simulink model "BLDCmotor_FOC_R2017b_fixdt"  (R2025a)
settings: Solver=FixedStepDiscrete  StartTime=0  StopTime=0.5  FixedStep=Ts  MaxStep=1e-6  RelTol=1e-6  AbsTol=1e-6  EnableMultiTasking=on
PreLoadFcn:
  | addpath(pwd);
  | addpath(genpath('01_Libraries'));
  | addpath(genpath('02_Figures'));
  | addpath(genpath('03_CreateParamTable'));
InitFcn:
  | init_model;
values from neighbouring files (symbols this model uses):
  a_cpr = 65535    [init_model.m]
  a_elecAngle = 60    [init_model.m]
  a_elecoffset = a_elecPeriod/12    (= 30)    [init_model.m]
  a_elecPeriod = 360    [init_model.m]
  a_fcpr = 1/65535    (= 1.52590218967e-05)    [init_model.m]
  a_mechoffset = a_elecoffset/n_polePairs    (= 5)    [init_model.m]
  a_phaAdvMax = 25    [init_model.m]
  b_angleMeasEna = 1    [init_model.m]
  b_cruiseCtrlEna = 0    [init_model.m]
  b_diagEna = 0    [init_model.m]
  b_fieldWeakEna = 0    [init_model.m]
  cf_currFilt = 0.692    [init_model.m]
  cf_idKi = Ki / (f_ctrl)    (= 0.00409061543436)    [init_model.m]
  cf_idKp = Kp    (= 0.0523598775598)    [init_model.m]
  cf_iqKi = Ki / (f_ctrl)    (= 0.00409061543436)    [init_model.m]
  cf_iqKiLimProt = 60 / (f_ctrl)    (= 0.00375)    [init_model.m]
  cf_iqKp = Kp    (= 0.0523598775598)    [init_model.m]
  cf_KbLimProt = Simulink.Parameter    [init_model.m]
  cf_nKi = 20.4 / (f_ctrl)    (= 0.001275)    [init_model.m]
  cf_nKiLimProt = 20 / (f_ctrl)    (= 0.00125)    [init_model.m]
  cf_nKp = 1.18    [init_model.m]
  cf_speedCoef = round(f_ctrl * a_mechAngle * (pi/180) * (30/pi))    [init_model.m]
  CTRL_FOC = 2    [init_model.m]
  CTRL_SIN = 1    [init_model.m]
  dV_openRate = 1000 / (f_ctrl)    (= 0.0625)    [init_model.m]
  dz_cntTrnsDetHi = 40    [init_model.m]
  dz_cntTrnsDetLo = 20    [init_model.m]
  ff_gain = ((r_motn / i_sca) * ((GD32_Vd_max_margin) / v_bus))    (= 0.338958333333)    [init_model.m]
  GD32_Vd_max_margin = GD32_Vd_max - V_margin    (= 1627)    [init_model.m]
  GD32_Vq_max_M1 = sqrt(GD32_Vd_max_margin^2 - GD32_Vq_max_XA.^2)    [init_model.m]
  i_max = i_max * i_sca    (= 500)    [init_model.m]
  id_fieldWeakMax = 5 * i_sca    (= 250)    [init_model.m]
  iq_maxSca_M1 = sqrt(1 - iq_maxSca_XA.^2)    [init_model.m]
  mcu_model = GD32F103    (= 1)    [init_model.m]
  n_commAcvLo = 15    [init_model.m]
  n_commDeacvHi = 30    [init_model.m]
  n_cruiseMotTgt = 0    [init_model.m]
  n_fieldWeakAuthHi = 300    [init_model.m]
  n_fieldWeakAuthLo = 100    [init_model.m]
  n_max = 1950    [init_model.m]
  n_polePairs = 6    [init_model.m]
  n_stdStillDet = 3    [init_model.m]
  OPEN_MODE = 0    [init_model.m]
  r_cos_M1 = cos((a_elecAngle_XA + a_elecPeriod/12)*(pi/180))    [init_model.m]
  r_errInpTgtThres = 600    [init_model.m]
  r_fieldWeakHi = 1000    [init_model.m]
  r_fieldWeakLo = 750    [init_model.m]
  r_motn = r_mot/2    (= 0.25)    [init_model.m]
  r_sin3PhaA_M1 = sin3Arm + A*r_sinPhaA_M1    [init_model.m]
  r_sin3PhaB_M1 = sin3Arm + A*r_sinPhaB_M1    [init_model.m]
  r_sin3PhaC_M1 = sin3Arm + A*r_sinPhaC_M1    [init_model.m]
  r_sin_M1 = sin((a_elecAngle_XA + a_elecPeriod/12)*(pi/180))    [init_model.m]
  SPD_MODE = 2    [init_model.m]
  STM32_Vd_max_margin = STM32_Vd_max - V_margin    (= 940)    [init_model.m]
  STM32_Vq_max_M1 = sqrt(STM32_Vd_max_margin^2 - STM32_Vq_max_XA.^2)    [init_model.m]
  t_errDequal = 1.80 * f_ctrl    (= 28800)    [init_model.m]
  t_errQual = 0.24 * f_ctrl    (= 3840)    [init_model.m]
  tgt_scale = 2047    [init_model.m]
  TRQ_MODE = 3    [init_model.m]
  Ts = 5e-6    (= 5e-06)    [init_model.m]
  Ts_ctrl = 6e-5    (= 6e-05)    [init_model.m]
  v_bus = 24    [init_model.m]
  vec_hallToPos = [0 2 0 1 4 3 5 0]    [init_model.m]
  VLT_MODE = 1    [init_model.m]
  z_commutMap_M1 = [-1 -1  0  1  1  0 ... (first row only)    [init_model.m]
  z_ctrlModReq = TRQ_MODE    (= 3)    [init_model.m]
  z_ctrlTypSel = CTRL_FOC    (= 2)    [init_model.m]
  z_maxCntRst = 2000    [init_model.m]
  z_selPhaCurMeasABC = 2    [init_model.m]
undefined symbols (not defined in the file or in its folder): BLDCmotor_FOC_R2017b_fixdt, DiscIntNeverNeededParam, DWORK0, DWORK1, DWORK2, DWORK3, powergui, spspowerguiLib
libraries: BLDC_controller_Lib x18, simulink x13, prociolib x6, eePwmGenerator x6, eePwmGeneratorMultilevel x3, mcbpositiondecoderlib x2, slpidlib x2, spsControlledVoltageSourceLib x1, spsMultimeterLib x1, spsPermanentMagnetSynchronousMachineLib x1, spsUniversalBridgeLib x1, spsVoltageMeasurementLib x1
(part 6 of 6)

== system BLDCmotor_FOC_R2017b_fixdt/BLDC_controller/F05_Field_Oriented_Control/FOC/FOC_Enabled/Torque_Mode/PI_clamp_fixdtFF ==
  err : Inport
  P : Inport  Port=2
  I : Inport  Port=3
  init : Inport  Port=4
  satMax : Inport  Port=5
  satMin : Inport  Port=6
  ext_limProt : Inport  Port=7
  FeedForward : Inport  Port=8
  AND1 : Logic  DisableCoverage=on  Operator=OR  OutDataTypeStr=boolean
  Clamping_circuit : Subsystem
  Constant : Constant  Value=0  OutDataTypeStr=Inherit: Inherit via back propagation
  Divide2 : Product  Inputs=**  RndMeth=Simplest
  Divide5 : Product  Inputs=**  OutDataTypeStr=fixdt(1,16,5)  RndMeth=Simplest  SaturateOnIntegerOverflow=on
  Input : Constant  Value=ff_gain  OutDataTypeStr=fixdt(1,16,12)
  Integrator : Subsystem
  Product : Product  OutDataTypeStr=fixdt(1,16,4)  SaturateOnIntegerOverflow=on
  Saturation_hit : BLDC_controller_Lib/Saturation_hit  SystemSampleTime=-1  VariantActivationTime=update diagram  EmptyChoice=off  PassThrough=off  PassThroughVariantControl=(default)  EmptyChoiceVariantControl=(default)  AllowFlexibleInterface=on  Latency=0  AutoFrameSizeCalculation=off
  Sum1 : Sum  OutDataTypeStr=fixdt(1,16,4)  RndMeth=Simplest  SaturateOnIntegerOverflow=on
  Sum2 : Sum  RndMeth=Simplest  SaturateOnIntegerOverflow=on
  Sum3 : Sum  Inputs=|++  OutDataTypeStr=fixdt(1,16,4)  SaturateOnIntegerOverflow=on
  Switch1 : Switch  Criteria=u2 ~= 0  OutDataTypeStr=Inherit: Inherit via back propagation  RndMeth=Zero  SaturateOnIntegerOverflow=off  InputSameDT=off
  UnitDelay1 : UnitDelay  SampleTime=-1  HasFrameUpgradeWarning=on
      settings: AttributesFormatString=Ini=%<X0>
  out : Outport  VectorParamsAs1DForOutWhenUnconnected=off
  wires:
  I/1 -> Divide2/2
  Sum2/1 -> Switch1/3, Clamping_circuit/1(preIntegrator)
  Sum3/1 -> Saturation_hit/2
  [b_hitSat] -> Clamping_circuit/3(hitSat)
  Saturation_hit/3 -> [b_hitMin]
  P/1 -> Divide5/2
  Saturation_hit/2 -> out/1
  [b_hitMin] -> AND1/2
  init/1 -> Integrator/2(init)
  UnitDelay1/1 -> Switch1/2
  Product/1 -> Sum3/1
  Divide5/1 -> Sum1/1
  satMax/1 -> Saturation_hit/1
  Clamping_circuit/1(Clamp) -> UnitDelay1/1
  FeedForward/1 -> Product/2
  err/1 -> Divide2/1, Divide5/1
  Constant/1 -> Switch1/1
  Saturation_hit/1 -> [b_hitMax]
  Sum1/1 -> Clamping_circuit/2(preSat), Sum3/2
  [b_hitMax] -> AND1/1
  satMin/1 -> Saturation_hit/3
  AND1/1 -> [b_hitSat]
  Switch1/1 -> Integrator/1(u)
  ext_limProt/1 -> Sum2/2
  Divide2/1 -> Sum2/1
  Integrator/1(y) -> Sum1/2
  Input/1 -> Product/1

== system BLDCmotor_FOC_R2017b_fixdt/BLDC_controller/F05_Field_Oriented_Control/FOC/FOC_Enabled/Torque_Mode/Variant Subsystem ==
  note: 1) Add Subsystem or Model blocks as valid variant choices.
      | 2) You cannot connect blocks at this level. At simulation, connectivity is automatically
      | determined, based on the active variant and port name matching.
  GD32F103 : Subsystem  TreatAsAtomicUnit=on  VariantControl=mcu_model == 1
  STM32F103 : Subsystem  TreatAsAtomicUnit=on  VariantControl=mcu_model == 0
  Vd_max_margin : Outport

== system BLDCmotor_FOC_R2017b_fixdt/BLDC_controller/F05_Field_Oriented_Control/FOC/FOC_Enabled/Vd_Calculation/PI_clamp_fixdtFF ==
  err : Inport
  P : Inport  Port=2
  I : Inport  Port=3
  init : Inport  Port=4
  satMax : Inport  Port=5
  satMin : Inport  Port=6
  ext_limProt : Inport  Port=7
  FeedForward : Inport  Port=8
  AND1 : Logic  DisableCoverage=on  Operator=OR  OutDataTypeStr=boolean
  Clamping_circuit : Subsystem
  Constant : Constant  Value=0  OutDataTypeStr=Inherit: Inherit via back propagation
  Divide2 : Product  Inputs=**  RndMeth=Simplest
  Divide5 : Product  Inputs=**  OutDataTypeStr=fixdt(1,16,5)  RndMeth=Simplest  SaturateOnIntegerOverflow=on
  Input : Constant  Value=ff_gain  OutDataTypeStr=fixdt(1,16,12)
  Integrator : Subsystem
  Product : Product  OutDataTypeStr=fixdt(1,16,4)  SaturateOnIntegerOverflow=on
  Saturation_hit : BLDC_controller_Lib/Saturation_hit  SystemSampleTime=-1  VariantActivationTime=update diagram  EmptyChoice=off  PassThrough=off  PassThroughVariantControl=(default)  EmptyChoiceVariantControl=(default)  AllowFlexibleInterface=on  Latency=0  AutoFrameSizeCalculation=off
  Sum1 : Sum  OutDataTypeStr=fixdt(1,16,4)  RndMeth=Simplest  SaturateOnIntegerOverflow=on
  Sum2 : Sum  RndMeth=Simplest  SaturateOnIntegerOverflow=on
  Sum3 : Sum  Inputs=|++  OutDataTypeStr=fixdt(1,16,4)  SaturateOnIntegerOverflow=on
  Switch1 : Switch  Criteria=u2 ~= 0  OutDataTypeStr=Inherit: Inherit via back propagation  RndMeth=Zero  SaturateOnIntegerOverflow=off  InputSameDT=off
  UnitDelay1 : UnitDelay  SampleTime=-1  HasFrameUpgradeWarning=on
      settings: AttributesFormatString=Ini=%<X0>
  out : Outport  VectorParamsAs1DForOutWhenUnconnected=off
  wires:
  I/1 -> Divide2/2
  Sum2/1 -> Switch1/3, Clamping_circuit/1(preIntegrator)
  Sum3/1 -> Saturation_hit/2
  [b_hitSat] -> Clamping_circuit/3(hitSat)
  Saturation_hit/3 -> [b_hitMin]
  P/1 -> Divide5/2
  Saturation_hit/2 -> out/1
  [b_hitMin] -> AND1/2
  init/1 -> Integrator/2(init)
  UnitDelay1/1 -> Switch1/2
  Divide5/1 -> Sum1/1
  satMax/1 -> Saturation_hit/1
  Clamping_circuit/1(Clamp) -> UnitDelay1/1
  err/1 -> Divide2/1, Divide5/1
  Constant/1 -> Switch1/1
  Saturation_hit/1 -> [b_hitMax]
  Sum1/1 -> Clamping_circuit/2(preSat), Sum3/2
  [b_hitMax] -> AND1/1
  satMin/1 -> Saturation_hit/3
  AND1/1 -> [b_hitSat]
  Switch1/1 -> Integrator/1(u)
  ext_limProt/1 -> Sum2/2
  Divide2/1 -> Sum2/1
  Integrator/1(y) -> Sum1/2
  FeedForward/1 -> Product/2
  Product/1 -> Sum3/1
  Input/1 -> Product/1

== system BLDCmotor_FOC_R2017b_fixdt/BLDC_controller/F05_Field_Oriented_Control/Motor_Limitations/Motor_Limitations_Enabled/Torque_Mode_Protection/Variant Subsystem1 ==
  note: 1) Add Subsystem or Model blocks as valid variant choices.
      | 2) You cannot connect blocks at this level. At simulation, connectivity is automatically
      | determined, based on the active variant and port name matching.
  GD32F103 : Subsystem  TreatAsAtomicUnit=on  VariantControl=mcu_model == 1
  STM32F103 : Subsystem  TreatAsAtomicUnit=on  VariantControl=mcu_model == 0
  Vd_max_margin : Outport

== system BLDCmotor_FOC_R2017b_fixdt/BLDC_controller/F05_Field_Oriented_Control/Motor_Limitations/Motor_Limitations_Enabled/Variant Subsystem/GD32F103 ==
  note: Voltage Circle limitations with priority on i_d (Flux current):
      | Vq_max = sqrt(Vd_max^2 - Vd^2)
      | Vq_min = -Vq_max
  VdPrev : Inport
  Abs5 : Abs  OutDataTypeStr=Inherit: Inherit via back propagation  RndMeth=Zero  SaturateOnIntegerOverflow=off
  Constant : Constant  Value=0  OutDataTypeStr=uint8
  GD32_Vq_max_M1 : Interpolation_n-D  NumberOfTableDimensions=1  Table=GD32_Vq_max_M1  InterpMethod=Flat  ExtrapMethod=Clip  DiagnosticForOutOfRangeInput=Error  RemoveProtectionIndex=on  ValidIndexMayReachLast=on  OutDataTypeStr=Inherit: Inherit via back propagation  InternalRulePriority=Speed  RndMeth=Simplest
      settings: InputPortMap=u0,u1
  GD32_Vq_max_XA : PreLookup  BreakpointsData=GD32_Vq_max_XA  OutputSelection=Index only  IndexSearchMethod=Evenly spaced points  BeginIndexSearchUsingPreviousIndexResult=on  UseLastBreakpoint=on  RemoveProtectionInput=on  IndexDataTypeStr=uint8  FractionDataTypeStr=fixdt(0,8,6)  RndMeth=Simplest
  Gain3 : Gain  Tag=struct('comment',struct('text','','placement',1),'logdata',struct('maxnumvals',inf,'plotchannels',[],'loggingmode',3,'channels',1),'output',struct('variable','','description','','name','$S_$B','width',1,'address','','max',NaN,'min',NaN,'class','default','type','CONTINUOUS','scaling','','lsb',1,'offset',0,'arb',0,'freeze',1,'unit','','autoscalingmode',1,'lowerheadroom',1,'upperheadroom',1,'headroomunit','bit','keepdatatype',1,'checkmin',0,'checkmax',0,'castoutput',0,'show',0),'gain',struct('variable','','description','','name','$S_$B_gain','width',1,'address','','max',NaN,'min',NaN,'class','default','type','CONTINUOUS','scaling','','lsb',1,'offset',0,'arb',0,'freeze',1,'unit','','keepdatatype',1,'value','1','scalar',0,'tolerance',1),'scalingvalid',0,'date',730486)  Gain=-1  RndMeth=Zero  OutDataTypeStr=Inherit: Same as input  ParamDataTypeStr=Inherit: Same as input
  Gain5 : Gain  Tag=struct('comment',struct('text','','placement',1),'logdata',struct('maxnumvals',inf,'plotchannels',[],'loggingmode',3,'channels',1),'output',struct('variable','','description','','name','$S_$B','width',1,'address','','max',NaN,'min',NaN,'class','default','type','CONTINUOUS','scaling','','lsb',1,'offset',0,'arb',0,'freeze',1,'unit','','autoscalingmode',1,'lowerheadroom',1,'upperheadroom',1,'headroomunit','bit','keepdatatype',1,'checkmin',0,'checkmax',0,'castoutput',0,'show',0),'gain',struct('variable','','description','','name','$S_$B_gain','width',1,'address','','max',NaN,'min',NaN,'class','default','type','CONTINUOUS','scaling','','lsb',1,'offset',0,'arb',0,'freeze',1,'unit','','keepdatatype',1,'value','1','scalar',0,'tolerance',1),'scalingvalid',0,'date',730486)  Gain=-1  RndMeth=Zero  OutDataTypeStr=Inherit: Same as input  ParamDataTypeStr=Inherit: Same as input
  Vd_max1 : Constant  Value=GD32_Vd_max_margin  OutDataTypeStr=fixdt(1,16,4)
  Vd_max : Outport
  Vq_min : Outport  Port=2
  Vq_max : Outport  Port=3
  Vd_min : Outport  Port=4
  wires:
  [VdPrev] -> Abs5/1
  Abs5/1 -> GD32_Vq_max_XA/1
  Vd_max1/1 -> Gain3/1, [Vd_max]
  VdPrev/1 -> [VdPrev]
  GD32_Vq_max_XA/1 -> GD32_Vq_max_M1/1
  [Vd_max] -> Vd_max/1
  [Vq_max] -> Vq_max/1
  Gain3/1 -> [Vd_min]
  Gain5/1 -> [Vq_min]
  [Vq_min] -> Vd_min/1
  GD32_Vq_max_M1/1 -> Gain5/1, [Vq_max]
  [Vd_min] -> Vq_min/1
  Constant/1 -> GD32_Vq_max_M1/2

== system BLDCmotor_FOC_R2017b_fixdt/BLDC_controller/F05_Field_Oriented_Control/Motor_Limitations/Motor_Limitations_Enabled/Variant Subsystem/STM32F103 ==
  note: Voltage Circle limitations with priority on i_d (Flux current):
      | Vq_max = sqrt(Vd_max^2 - Vd^2)
      | Vq_min = -Vq_max
  VdPrev : Inport
  Abs5 : Abs  OutDataTypeStr=Inherit: Inherit via back propagation  RndMeth=Zero  SaturateOnIntegerOverflow=off
  Constant : Constant  Value=0  OutDataTypeStr=uint8
  Gain3 : Gain  Tag=struct('comment',struct('text','','placement',1),'logdata',struct('maxnumvals',inf,'plotchannels',[],'loggingmode',3,'channels',1),'output',struct('variable','','description','','name','$S_$B','width',1,'address','','max',NaN,'min',NaN,'class','default','type','CONTINUOUS','scaling','','lsb',1,'offset',0,'arb',0,'freeze',1,'unit','','autoscalingmode',1,'lowerheadroom',1,'upperheadroom',1,'headroomunit','bit','keepdatatype',1,'checkmin',0,'checkmax',0,'castoutput',0,'show',0),'gain',struct('variable','','description','','name','$S_$B_gain','width',1,'address','','max',NaN,'min',NaN,'class','default','type','CONTINUOUS','scaling','','lsb',1,'offset',0,'arb',0,'freeze',1,'unit','','keepdatatype',1,'value','1','scalar',0,'tolerance',1),'scalingvalid',0,'date',730486)  Gain=-1  RndMeth=Zero  OutDataTypeStr=Inherit: Same as input  ParamDataTypeStr=Inherit: Same as input
  Gain5 : Gain  Tag=struct('comment',struct('text','','placement',1),'logdata',struct('maxnumvals',inf,'plotchannels',[],'loggingmode',3,'channels',1),'output',struct('variable','','description','','name','$S_$B','width',1,'address','','max',NaN,'min',NaN,'class','default','type','CONTINUOUS','scaling','','lsb',1,'offset',0,'arb',0,'freeze',1,'unit','','autoscalingmode',1,'lowerheadroom',1,'upperheadroom',1,'headroomunit','bit','keepdatatype',1,'checkmin',0,'checkmax',0,'castoutput',0,'show',0),'gain',struct('variable','','description','','name','$S_$B_gain','width',1,'address','','max',NaN,'min',NaN,'class','default','type','CONTINUOUS','scaling','','lsb',1,'offset',0,'arb',0,'freeze',1,'unit','','keepdatatype',1,'value','1','scalar',0,'tolerance',1),'scalingvalid',0,'date',730486)  Gain=-1  RndMeth=Zero  OutDataTypeStr=Inherit: Same as input  ParamDataTypeStr=Inherit: Same as input
  STM32_Vq_max_M1 : Interpolation_n-D  NumberOfTableDimensions=1  Table=STM32_Vq_max_M1  InterpMethod=Flat  ExtrapMethod=Clip  DiagnosticForOutOfRangeInput=Error  RemoveProtectionIndex=on  ValidIndexMayReachLast=on  OutDataTypeStr=fixdt(1,16,4)  InternalRulePriority=Speed  RndMeth=Simplest
      settings: InputPortMap=u0,u1
  STM32_Vq_max_XA : PreLookup  BreakpointsData=STM32_Vq_max_XA  OutputSelection=Index only  IndexSearchMethod=Evenly spaced points  BeginIndexSearchUsingPreviousIndexResult=on  UseLastBreakpoint=on  RemoveProtectionInput=on  IndexDataTypeStr=uint8  FractionDataTypeStr=fixdt(0,8,6)  RndMeth=Simplest
  Vd_max2 : Constant  Value=STM32_Vd_max_margin  OutDataTypeStr=fixdt(1,16,4)
  Vd_max : Outport
  Vq_min : Outport  Port=2
  Vq_max : Outport  Port=3
  Vd_min : Outport  Port=4
  wires:
  Abs5/1 -> STM32_Vq_max_XA/1
  STM32_Vq_max_XA/1 -> STM32_Vq_max_M1/1
  [Vd_max] -> Vd_max/1
  [Vq_max] -> Vq_max/1
  VdPrev/1 -> [VdPrev]
  [VdPrev] -> Abs5/1
  Gain5/1 -> [Vq_min]
  STM32_Vq_max_M1/1 -> Gain5/1, [Vq_max]
  [Vq_min] -> Vd_min/1
  Vd_max2/1 -> Gain3/1, [Vd_max]
  [Vd_min] -> Vq_min/1
  Gain3/1 -> [Vd_min]
  Constant/1 -> STM32_Vq_max_M1/2

== system BLDCmotor_FOC_R2017b_fixdt/BLDC_controller/F05_Field_Oriented_Control/FOC/FOC_Enabled/Torque_Mode/PI_clamp_fixdtFF/Clamping_circuit ==
  preIntegrator : Inport  DisableCoverage=on
  preSat : Inport  DisableCoverage=on  Port=2
  hitSat : Inport  DisableCoverage=on  Port=3
  AND1 : Logic  DisableCoverage=on  OutDataTypeStr=boolean
  DataTypeConv3 : DataTypeConversion  DisableCoverage=on  OutDataTypeStr=int8  SaturateOnIntegerOverflow=off  LockScale=on
  DataTypeConv4 : DataTypeConversion  DisableCoverage=on  OutDataTypeStr=int8  SaturateOnIntegerOverflow=off  LockScale=on
  Equal1 : RelationalOperator  DisableCoverage=on  Operator===  RndMeth=Zero
  SignDeltaU2 : Signum  DisableCoverage=on
  SignDeltaU3 : Signum  DisableCoverage=on
  Clamp : Outport  DisableCoverage=on  VectorParamsAs1DForOutWhenUnconnected=off
  wires:
  hitSat/1 -> AND1/2
  AND1/1 -> Clamp/1
  Equal1/1 -> AND1/1
  DataTypeConv4/1 -> Equal1/2
  DataTypeConv3/1 -> Equal1/1
  SignDeltaU3/1 -> DataTypeConv4/1
  SignDeltaU2/1 -> DataTypeConv3/1
  preSat/1 -> SignDeltaU3/1
  preIntegrator/1 -> SignDeltaU2/1

== system BLDCmotor_FOC_R2017b_fixdt/BLDC_controller/F05_Field_Oriented_Control/FOC/FOC_Enabled/Torque_Mode/PI_clamp_fixdtFF/Integrator ==
  u : Inport
  init : Inport  Port=2
  Data Type Conversion1 : DataTypeConversion  OutDataTypeStr=fixdt(1,16,4)  SaturateOnIntegerOverflow=off  RndMeth=Floor
  Resettable Delay : Delay  DelayLength=1  InitialConditionSource=Input port
      settings: InputPortMap=u0,p4
  Sum1 : Sum  Inputs=|++  RndMeth=Simplest  OutDataTypeStr=Inherit: Same as first input
  y : Outport  VectorParamsAs1DForOutWhenUnconnected=off
  wires:
  init/1 -> Resettable Delay/2
  Data Type Conversion1/1 -> y/1
  Resettable Delay/1 -> Sum1/2
  Sum1/1 -> Data Type Conversion1/1, Resettable Delay/1
  u/1 -> Sum1/1

== system BLDCmotor_FOC_R2017b_fixdt/BLDC_controller/F05_Field_Oriented_Control/FOC/FOC_Enabled/Torque_Mode/Variant Subsystem/GD32F103 ==
  Vd_max1 : Constant  Value=GD32_Vd_max_margin  OutDataTypeStr=fixdt(1,16,4)
  Vd_max_margin : Outport
  wires:
  Vd_max1/1 -> Vd_max_margin/1

== system BLDCmotor_FOC_R2017b_fixdt/BLDC_controller/F05_Field_Oriented_Control/FOC/FOC_Enabled/Torque_Mode/Variant Subsystem/STM32F103 ==
  Vd_max3 : Constant  Value=STM32_Vd_max_margin  OutDataTypeStr=fixdt(1,16,4)
  Vd_max_margin : Outport
  wires:
  Vd_max3/1 -> Vd_max_margin/1

== system BLDCmotor_FOC_R2017b_fixdt/BLDC_controller/F05_Field_Oriented_Control/FOC/FOC_Enabled/Vd_Calculation/PI_clamp_fixdtFF/Clamping_circuit ==
  preIntegrator : Inport  DisableCoverage=on
  preSat : Inport  DisableCoverage=on  Port=2
  hitSat : Inport  DisableCoverage=on  Port=3
  AND1 : Logic  DisableCoverage=on  OutDataTypeStr=boolean
  DataTypeConv3 : DataTypeConversion  DisableCoverage=on  OutDataTypeStr=int8  SaturateOnIntegerOverflow=off  LockScale=on
  DataTypeConv4 : DataTypeConversion  DisableCoverage=on  OutDataTypeStr=int8  SaturateOnIntegerOverflow=off  LockScale=on
  Equal1 : RelationalOperator  DisableCoverage=on  Operator===  RndMeth=Zero
  SignDeltaU2 : Signum  DisableCoverage=on
  SignDeltaU3 : Signum  DisableCoverage=on
  Clamp : Outport  DisableCoverage=on  VectorParamsAs1DForOutWhenUnconnected=off
  wires:
  hitSat/1 -> AND1/2
  AND1/1 -> Clamp/1
  Equal1/1 -> AND1/1
  DataTypeConv4/1 -> Equal1/2
  DataTypeConv3/1 -> Equal1/1
  SignDeltaU3/1 -> DataTypeConv4/1
  SignDeltaU2/1 -> DataTypeConv3/1
  preSat/1 -> SignDeltaU3/1
  preIntegrator/1 -> SignDeltaU2/1

== system BLDCmotor_FOC_R2017b_fixdt/BLDC_controller/F05_Field_Oriented_Control/FOC/FOC_Enabled/Vd_Calculation/PI_clamp_fixdtFF/Integrator ==
  u : Inport
  init : Inport  Port=2
  Data Type Conversion1 : DataTypeConversion  OutDataTypeStr=fixdt(1,16,4)  SaturateOnIntegerOverflow=off  RndMeth=Floor
  Resettable Delay : Delay  DelayLength=1  InitialConditionSource=Input port
      settings: InputPortMap=u0,p4
  Sum1 : Sum  Inputs=|++  RndMeth=Simplest  OutDataTypeStr=Inherit: Same as first input
  y : Outport  VectorParamsAs1DForOutWhenUnconnected=off
  wires:
  init/1 -> Resettable Delay/2
  Data Type Conversion1/1 -> y/1
  Resettable Delay/1 -> Sum1/2
  Sum1/1 -> Data Type Conversion1/1, Resettable Delay/1
  u/1 -> Sum1/1

== system BLDCmotor_FOC_R2017b_fixdt/BLDC_controller/F05_Field_Oriented_Control/Motor_Limitations/Motor_Limitations_Enabled/Torque_Mode_Protection/Variant Subsystem1/GD32F103 ==
  Vd_max1 : Constant  Value=GD32_Vd_max_margin  OutDataTypeStr=fixdt(1,16,4)
  Vd_max_margin : Outport
  wires:
  Vd_max1/1 -> Vd_max_margin/1

== system BLDCmotor_FOC_R2017b_fixdt/BLDC_controller/F05_Field_Oriented_Control/Motor_Limitations/Motor_Limitations_Enabled/Torque_Mode_Protection/Variant Subsystem1/STM32F103 ==
  Vd_max3 : Constant  Value=STM32_Vd_max_margin  OutDataTypeStr=fixdt(1,16,4)
  Vd_max_margin : Outport
  wires:
  Vd_max3/1 -> Vd_max_margin/1

== stateflow chart BLDCmotor_FOC_R2017b_fixdt/BLDC_controller/Task_Scheduler ==
  (default) -> (junction 9)
  (junction 9) -> (junction 11) [order 1] : [call1]{task1a; task1b;task3}
  (junction 9) -> (junction 13) [order 2]
  (junction 13) -> (junction 15) [order 1] : [call2]{task1b;task2a; task2b;task3}
  (junction 13) -> (junction 17) [order 2]
  (junction 17) -> (junction 19) : [call3]{task1b;task3}
  data: call1 input boolean; call2 input boolean; call3 input boolean
  events: task1a output FUNCTION_CALL_EVENT; task1b output FUNCTION_CALL_EVENT; task2a output FUNCTION_CALL_EVENT; task2b output FUNCTION_CALL_EVENT; task3 output FUNCTION_CALL_EVENT

== stateflow chart BLDCmotor_FOC_R2017b_fixdt/BLDC_controller/F03_Control_Mode_Manager/F03_02_Control_Mode_Manager ==
  state OPEN
    entry:
    z_ctrlMod = OPEN_MODE;
  state ACTIVE
    state TORQUE_MODE
      entry:
      z_ctrlMod = TRQ_MODE;
    state SPEED_MODE
      entry:
      z_ctrlMod = SPD_MODE;
    state VOLTAGE_MODE
      entry:
      z_ctrlMod = VLT_MODE;
    (default) -> (junction 7)
    TORQUE_MODE -> ACTIVE : [~b_toTrqMod]
    (junction 7) -> TORQUE_MODE [order 1] : [b_toTrqMod]
    (junction 7) -> (junction 8) [order 2]
    SPEED_MODE -> ACTIVE : [~b_toSpdMod]
    (junction 8) -> SPEED_MODE [order 1] : [b_toSpdMod]
    (junction 8) -> (junction 29) [order 2]
    VOLTAGE_MODE -> ACTIVE : [b_toTrqMod || ...
        | b_toSpdMod]
    (junction 29) -> VOLTAGE_MODE
  (default) -> OPEN
  OPEN -> ACTIVE : [b_toActive]
  ACTIVE -> OPEN : [b_toOpen]
  data: b_toOpen input boolean; b_toActive input boolean; b_toSpdMod input boolean; z_ctrlMod output uint8; OPEN_MODE constant uint8 =OPEN_MODE; TRQ_MODE constant uint8 =TRQ_MODE; SPD_MODE constant uint8 =SPD_MODE; VLT_MODE constant uint8 =VLT_MODE; b_toTrqMod input boolean
